simulink model "speed_controller"  (R2023b)
settings: Solver=VariableStepAuto  StartTime=0.0  StopTime=7  RelTol=1e-3
values from neighbouring files (symbols this model uses):
  Kds = 0    [Model_Vars.mat]    (also in pid_tuner.m = sys_pid.Kd)
  Kis = 518.460425454    [Model_Vars.mat]    (also in pid_tuner.m = sys_pid.Ki)
  Kps = 20.988816794    [Model_Vars.mat]    (also in pid_tuner.m = sys_pid.Kp)
undefined symbols (not defined in the file or in its folder): plecs, STire
libraries: nesl_utility x6, fl_lib x5, sdl_lib x3, slpidlib x1, vehdynlibtire x1
settings Model: Creator=jaz43  LastModifiedBy=jaz43
settings SolverCC: InitialStep=.0001  MaxConsecutiveMinStep=100
settings DebuggingCC: AlgebraicLoopMsg=none

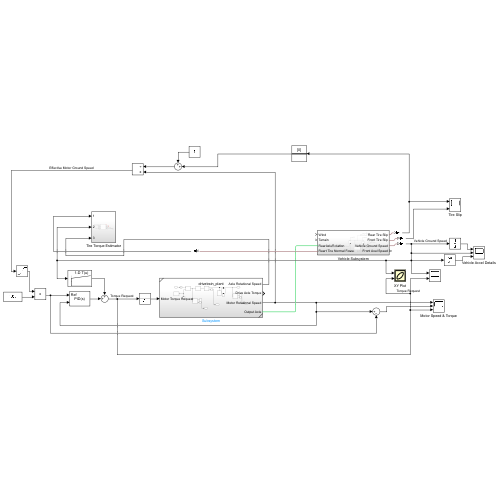
[thumbnail: Simulink's stored preview of the top-level diagram]
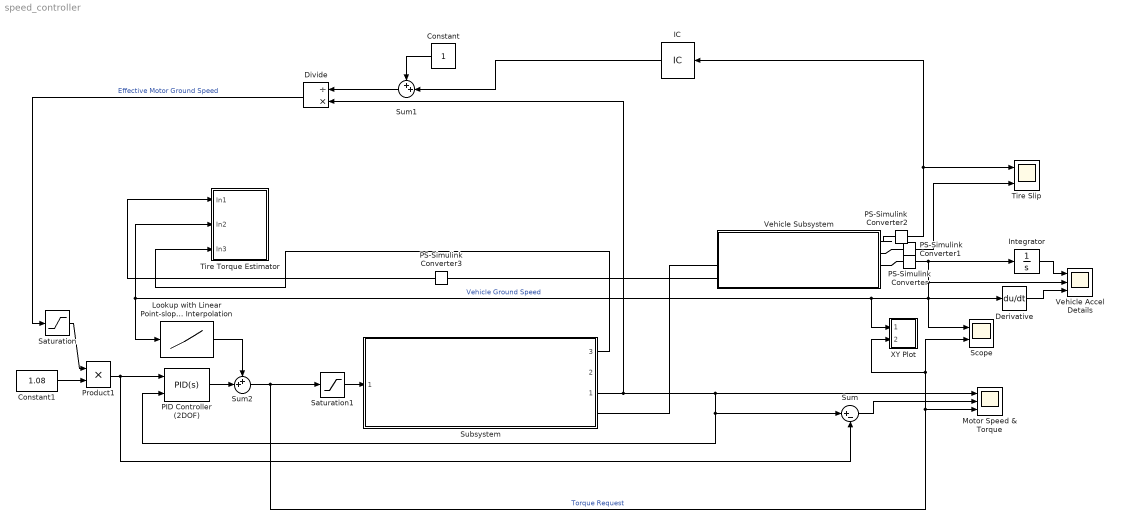
== system speed_controller ==
  Constant : Constant
  Constant1 : Constant  Value=1.08
  Derivative : Derivative
  Divide : Product  Inputs=/*
  IC : InitialCondition  Value=0
  Integrator : Integrator
  Lookup with Linear Point-slope Interpolation : Lookup_n-D  NumberOfTableDimensions=1  BreakpointsForDimension1=[0;0.02;0.05;0.1;0.5;60]  Table=[185;185;185;200;210;218]  InternalRulePriority=Speed  RndMeth=Simplest
  Motor Speed & Torque : Scope  NumInputPorts=3
  PID Controller (2DOF) : slpidlib/PID Controller (2DOF)  Controller=PID  Form=Parallel  TimeDomain=Continuous-time  UseExternalTs=off  SampleTime=-1  IntegratorMethod=Forward Euler  FilterMethod=Forward Euler  ControllerParametersSource=internal  P=Kps  I=Kis  UseKiTs=off  D=Kds  N=0  UseFilter=on  b=1  c=1  TunerSelectOption=Transfer Function Based (PID Tuner App)  InitialConditionSource=internal  InitialConditionForIntegrator=0  InitialConditionForFilter=0  DifferentiatorICPrevScaledInput=0  ExternalReset=none  TrackingMode=off  Kt=1  LimitOutput=off  SatLimitsSource=internal  UpperSaturationLimit=inf  LowerSaturationLimit=-inf  LinearizeAsGain=on  AntiWindupMode=none  Kb=1  LimitIntegrator=on  UpperIntegratorSaturationLimit=20  LowerIntegratorSaturationLimit=-20  POutMin=[]  POutMax=[]  IOutMin=[]  IOutMax=[]  DOutMin=[]  DOutMax=[]  NOutMin=[]  NOutMax=[]  bOutMin=[]  bOutMax=[]  cOutMin=[]  cOutMax=[]  SumOutMin=[]  SumOutMax=[]  SaturationOutMin=[]  SaturationOutMax=[]  PParamMin=[]  PParamMax=[]  IParamMin=[]  IParamMax=[]  DParamMin=[]  DParamMax=[]  NParamMin=[]  NParamMax=[]  bParamMin=[]  bParamMax=[]  cParamMin=[]  cParamMax=[]  KbParamMin=[]  KbParamMax=[]  KtParamMin=[]  KtParamMax=[]  KbOutMin=[]  KbOutMax=[]  KtOutMin=[]  KtOutMax=[]  IntegratorOutMin=[]  IntegratorOutMax=[]  FilterOutMin=[]  FilterOutMax=[]  SumI1OutMin=[]  SumI1OutMax=[]  SumI2OutMin=[]  SumI2OutMax=[]  SumI3OutMin=[]  SumI3OutMax=[]  SumI4OutMin=[]  SumI4OutMax=[]  SumDOutMin=[]  SumDOutMax=[]  Sum1OutMin=[]  Sum1OutMax=[]  Sum2OutMin=[]  Sum2OutMax=[]  Sum3OutMin=[]  Sum3OutMax=[]  DifferentiatorOutMin=[]  DifferentiatorOutMax=[]  FilterDiffOutCoefMin=[]  FilterDiffOutCoefMax=[]  ReciprocalOutMin=[]  ReciprocalOutMax=[]  SumDenOutMin=[]  SumDenOutMax=[]  SumNumOutMin=[]  SumNumOutMax=[]  DivideOutMin=[]  DivideOutMax=[]  UdiffTsProdOutMin=[]  UdiffTsProdOutMax=[]  NTsProdOutMin=[]  NTsProdOutMax=[]  UintegralTsProdOutMin=[]  UintegralTsProdOutMax=[]  UngainTsProdOutMin=[]  UngainTsProdOutMax=[]  ClampingZeroOutDataTypeStr=Inherit: Inherit via back propagation  ClampingZeroOutMin=[]  ClampingZeroOutMax=[]  FilterDenConstantOutDataTypeStr=Inherit: Inherit via back propagation  FilterDenConstantOutMin=[]  FilterDenConstantOutMax=[]  PCopyOutDataTypeStr=Inherit: Inherit via back propagation  PCopyOutMin=[]  PCopyOutMax=[]  NCopyOutDataTypeStr=Inherit: Inherit via back propagation  NCopyOutMin=[]  NCopyOutMax=[]  IntegratorContinuousStateAttributes=''  IntegratorStateMustResolveToSignalObject=off  IntegratorRTWStateStorageClass=Auto  FilterContinuousStateAttributes=''  FilterStateMustResolveToSignalObject=off  FilterRTWStateStorageClass=Auto  ParallelPVariant=InternalParameters  IdealPVariant=Disabled  IVariant=InternalParameters  DVariant=InternalParameters  bVariant=InternalParameters  cVariant=InternalParameters  IntegratorVariant=Continuous  SatVariant=Disabled  AWVariant=Passthrough  PCopyVariant=Disabled  TRVariant=Disabled  FdbkBlocksVariant=Forward  IdealPFdbkVariant=Disabled  SatFdbkVariant=Disabled  DerivativeFilterVariant=ContFilter  NVariant=InternalParameters  NCopyVariant=Disabled  FilterICVariant=InternalICsFilter  IntegratorICVariant=InternalICs  ExternalResetVariant=Disabled  TRSumVariant=Passthrough  SumFdbkVariant=Disabled  SumVariant=Sum_PID  TsampFilterVariant=InternalTs  TsampNgainVariant=Passthrough  TsampIntegralVariant=Disabled_SignalSpec  ExternalSaturationOutDataTypeStr=Inherit: Same as second input
  PS-Simulink Converter : nesl_utility/PS-Simulink Converter  PhysicalDomain=network_engine_domain  SubClassName=ps_output  LeftPortType=input  RightPortType=output  PseudoPeriodic=off  Frequencies=[]  VectorFormat=inherit  Unit=m/s  AffineConversion=off
  PS-Simulink Converter1 : nesl_utility/PS-Simulink Converter  PhysicalDomain=network_engine_domain  SubClassName=ps_output  LeftPortType=input  RightPortType=output  PseudoPeriodic=off  Frequencies=[]  VectorFormat=inherit  Unit=inherit  AffineConversion=off
  PS-Simulink Converter2 : nesl_utility/PS-Simulink Converter  PhysicalDomain=network_engine_domain  SubClassName=ps_output  LeftPortType=input  RightPortType=output  PseudoPeriodic=off  Frequencies=[]  VectorFormat=inherit  Unit=inherit  AffineConversion=off
  PS-Simulink Converter3 : nesl_utility/PS-Simulink Converter  PhysicalDomain=network_engine_domain  SubClassName=ps_output  LeftPortType=input  RightPortType=output  PseudoPeriodic=off  Frequencies=[]  VectorFormat=inherit  Unit=N  AffineConversion=off
  Product1 : Product
  Saturation : Saturate  UpperLimit=10000  LowerLimit=.2
  Saturation1 : Saturate  UpperLimit=230  LowerLimit=-15
  Scope : Scope  NumInputPorts=2
  Subsystem : Subsystem  ReferencedSubsystem=drivetrain_plant
      settings: PortSchema="{\"entries\":[{\"content\":{\"sides\":[{\"content\":{\"connectorIds\":[\"In1\"]},\"type\":\"ConnectorPlacement.EquallySpacedRectSide\",\"uuid\":\"fd89c741-3730-40e8-897c-6a9596430380\"},{\"content\":{\"connectorIds\":[\"Out3\",\"Out2\",\"Out1\",\"RConn1\"],\"side\":\"RIGHT\"},\"type\":\"ConnectorPlacement.EquallySpacedRectSide\",\"uuid\":\"e89eb803-7163-4d37-b99f-28b08d4d828e\"},{\"content\":{\"side\":\"TOP\"},\"type\":\"ConnectorPlacement.EquallySpacedRectSide\",\"uuid\":\"f6f95d47-8b04-417b-a055-58bf5cd7e8eb\"}]},\"type\":\"ConnectorPlacement.EquallySpacedConnector\",\"uuid\":\"a2ebceaa-6fc6-457a-8fcb-4683c2947838\"}],\"packageUris\":[\"http://schema.mathworks.com/mf0/Connector/R2020b\"],\"version\":\"1.0\"}"
  Sum : Sum  Inputs=|+-
  Sum1 : Sum  Inputs=++|
  Sum2 : Sum  Inputs=++|
  Tire Slip : Scope  NumInputPorts=2
  Tire Torque Estimator : Subsystem
  Vehicle Accel Details : Scope  NumInputPorts=3
  Vehicle Subsystem : Subsystem
  XY Plot : Subsystem  LoadFcn=plecs('sl', 317);  InitFcn=plecs('sl', 314);  StartFcn=plecs('sl', 308);  StopFcn=plecs('sl', 309);  mask{Settings=<binary blob, 624 chars, not shown>}
      mask init:
      | plecs('sl', 315);
      settings: CopyFcn=plecs('sl', 318);  DeleteFcn=plecs('sl', 305);  UndoDeleteFcn=plecs('sl', 306);  PreSaveFcn=plecs('sl', 311);  NameChangeFcn=plecs('sl', 310);  DestroyFcn=plecs('sl', 307);  OpenFcn=plecs('sl', 302);  ErrorFcn=plerrorfcn
      mask Display:
      | plot([0.05 0.95 0.95 0.05 0.05], [0.95 0.95 0.05 0.05 0.95])
      | plot(0.5+sin((0:0.2:2)*pi)*0.3, 0.5+sin((0:0.2:2)*pi + pi/4)*0.3);
  wires:
  Sum/1 -> Motor Speed & Torque/2
  PS-Simulink Converter2/1 -> IC/1, Tire Slip/1
  PS-Simulink Converter1/1 -> Tire Slip/2
  Integrator/1 -> Vehicle Accel Details/1
  Derivative/1 -> Vehicle Accel Details/3
  Subsystem/1 -> Divide/2, PID Controller (2DOF)/2, Sum/1, Motor Speed & Torque/1
  Sum1/1 -> Divide/1
  Constant/1 -> Sum1/1
  Constant1/1 -> Product1/2
  Divide/1 -> Saturation/1  "Effective Motor Ground Speed"
  Saturation/1 -> Product1/1
  Sum2/1 -> Saturation1/1, XY Plot/2(2), Scope/2, Motor Speed & Torque/3  "Torque Request"
  PID Controller (2DOF)/1 -> Sum2/2
  IC/1 -> Sum1/2
  Product1/1 -> PID Controller (2DOF)/1, Sum/2
  PS-Simulink Converter/1 -> Derivative/1, Scope/1, XY Plot/1(1), Lookup with Linear Point-slope Interpolation/1, Tire Torque Estimator/2(In2), Vehicle Accel Details/2, Integrator/1  "Vehicle Ground Speed"
  PS-Simulink Converter3/1 -> Tire Torque Estimator/1(In1)
  Subsystem/3 -> Tire Torque Estimator/3(In3)
  Lookup with Linear Point-slope Interpolation/1 -> Sum2/1
  Saturation1/1 -> Subsystem/1
  connections:
  Subsystem/RConn1 -- Vehicle Subsystem/LConn3
  Vehicle Subsystem/RConn3 -- PS-Simulink Converter/LConn1
  PS-Simulink Converter1/LConn1 -- Vehicle Subsystem/RConn2
  Vehicle Subsystem/RConn1 -- PS-Simulink Converter2/LConn1
  Vehicle Subsystem/LConn4 -- PS-Simulink Converter3/LConn1

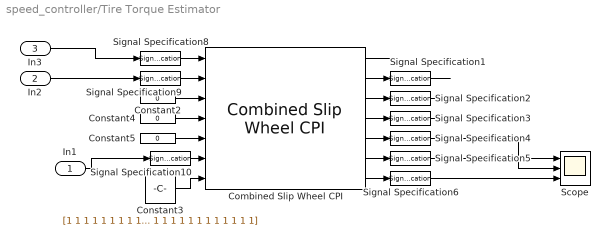
== system speed_controller/Tire Torque Estimator ==
  In1 : Inport
  In2 : Inport  Port=2
  In3 : Inport  Port=3
  Combined Slip Wheel CPI : vehdynlibtire/Combined Slip Wheel CPI  tireType=External file  tireParamSet=C:\Users\jaz43\Documents\2024\Projects\FSAE-LC\Simulink Car Model\testSimscapeCarModel\newtiremodel.tir  TireSide=Left  TirePrs=96526.6  extTirePrs=off  TireIO=CPI  plySteer=off  turnslip=off  PRESMAX=413685.6  PRESMIN=0  FZMAX=100000  FZMIN=0  VXLOW=1  KPUMAX=10  KPUMIN=-10  ALPMAX=0.523598775598299  ALPMIN=-0.523598775598299  CAMMAX=0.174532925199433  CAMMIN=-0.174532925199433  LONGVL=10  tyreside='Right'  FxRelFreqLwrLim=100*pi  FyRelFreqLwrLim=200*pi  MyRelFreqLwrLim=200*pi  omegao=0  br=1e-3  UNLOADED_RADIUS=0.3  NOMPRES=84000  FNOMIN=1500  WIDTH=0.2  RIM_RADIUS=0.2286  ASPECT_RATIO=3.5/6.9  MASS=.1  IYY=1.084  GRAVITY=-9.81  zo=0  zdoto=0  BREFF=8.39  DREFF=0.31475  FREFF=0.14694  Q_RE0=1.003  Q_V1=0.000864  Q_V2=0.025807  Q_FZ1=0  Q_FZ2=51.51  Q_FZ3=0  Q_FCX=0  Q_FCY=0  Q_FCY2=0  PFZ1=1  VERTICAL_STIFFNESS=283576.3  VERTICAL_DAMPING=500  BOTTOM_OFFST=0.01  BOTTOM_STIFF=2000000  Q_CAM1=0  Q_CAM2=0  Q_CAM3=0  LONGITUDINAL_STIFFNESS=505632.6  LATERAL_STIFFNESS=219162.7  PCFX1=-0.12193  PCFX2=0  PCFX3=0  PCFY1=-0.17034  PCFY2=0  PCFY3=0  Q_RA1=0.602  Q_RA2=1.024  Q_RB1=1.1137  Q_RB2=-0.09748  PCX1=1.9  PDX1=2  PDX2=-0.01  PDX3=10  PEX1=-1  PEX2=0.3  PEX3=0  PEX4=0  PKX1=20  PKX2=10  PKX3=0  PHX1=0  PHX2=0  PVX1=0  PVX2=0  PPX1=0  PPX2=0  PPX3=0  PPX4=0  RBX1=5  RBX2=5  RBX3=0  RCX1=1  REX1=-1  REX2=-0.1  RHX1=0  QSX1=0  QSX2=1.5  QSX3=0.1  QSX4=0.1  QSX5=0  QSX6=0  QSX7=0.1  QSX8=0  QSX9=0  QSX10=0  QSX11=0  QSX12=0  QSX13=0  QSX14=0  PPMX1=0  PCY1=2  PDY1=0.8  PDY2=-0.05  PDY3=0  PEY1=-0.8  PEY2=-0.6  PEY3=0.1  PEY4=0  PEY5=0  PKY1=-20  PKY2=2  PKY3=0  PKY4=2  PKY5=0  PKY6=0  PKY7=0  PHY1=0  PHY2=0  PVY1=0  PVY2=0  PVY3=0  PVY4=0  PPY1=0.1  PPY2=0.1  PPY3=0  PPY4=0  PPY5=0  RBY1=5  RBY2=2  RBY3=0.02  RBY4=0  RCY1=1  REY1=-0.1  REY2=0.1  RHY1=0  RHY2=0  RVY1=0  RVY2=0  RVY3=0  RVY4=0  RVY5=0  RVY6=0  QSY1=0  QSY2=0  QSY3=0  QSY4=0  QSY5=0  QSY6=0  QSY7=0  QSY8=0  QBZ1=2.2204e-16  QBZ2=0  QBZ3=0  QBZ4=0  QBZ5=0  QBZ6=0  QBZ9=0  QBZ10=0  QCZ1=0.1  QDZ1=0.1  QDZ2=0  QDZ3=0  QDZ4=0  QDZ6=0  QDZ7=0  QDZ8=0  QDZ9=0  QDZ10=0  QDZ11=0  QEZ1=0  QEZ2=0  QEZ3=0  QEZ4=0  QEZ5=0  QHZ1=0  QHZ2=0  QHZ3=0  QHZ4=0  PPZ1=0  PPZ2=0  SSZ1=0  SSZ2=0  SSZ3=0  SSZ4=0  PDXP1=0  PDXP2=0  PDXP3=0  PKYP1=0  PDYP1=0  PDYP2=0  PDYP3=0  PDYP4=0  PHYP1=0  PHYP2=0  PHYP3=0  PHYP4=0  PECP1=0  PECP2=0  QDTP1=0  QCRP1=0  QCRP2=0  QBRP1=0  QDRP1=0  QDRP2=0  aMode=2
  Constant2 : Constant  Value=0
  Constant3 : Constant  Value=[1 1 1 1 1 1 1 1 1 1 1 1 1 1 1 1 1 1 1 1 1 1 1 1 1 1 1]
  Constant4 : Constant  Value=0
  Constant5 : Constant  Value=0
  Scope : Scope  NumInputPorts=3
  Signal Specification{1..6,8..10} (9 alike) : SignalSpecification  Dimensions=1
  wires:
  Signal Specification4/1 -> Scope/2
  Signal Specification1/1 -> ?
  Signal Specification6/1 -> Scope/3
  Combined Slip Wheel CPI/3 -> Signal Specification2/1
  Combined Slip Wheel CPI/5 -> Signal Specification4/1
  Constant2/1 -> Combined Slip Wheel CPI/3
  Constant5/1 -> Combined Slip Wheel CPI/5
  Combined Slip Wheel CPI/2 -> Signal Specification1/1
  Signal Specification9/1 -> Combined Slip Wheel CPI/2
  Combined Slip Wheel CPI/6 -> Signal Specification5/1
  Signal Specification5/1 -> Scope/1
  Constant3/1 -> Combined Slip Wheel CPI/7
  Signal Specification8/1 -> Combined Slip Wheel CPI/1
  Constant4/1 -> Combined Slip Wheel CPI/4
  Combined Slip Wheel CPI/7 -> Signal Specification6/1
  Combined Slip Wheel CPI/1 -> ?
  Combined Slip Wheel CPI/4 -> Signal Specification3/1
  Signal Specification10/1 -> Combined Slip Wheel CPI/6
  In2/1 -> Signal Specification9/1
  In1/1 -> Signal Specification10/1
  In3/1 -> Signal Specification8/1
  Signal Specification3/1 -> ?
  Signal Specification2/1 -> ?

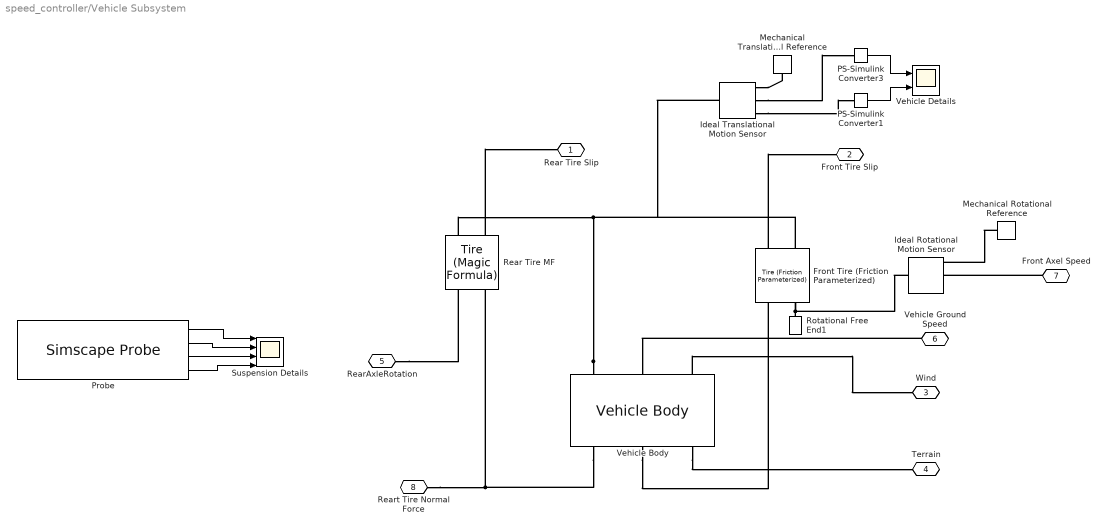
== system speed_controller/Vehicle Subsystem ==
  Front Tire (Friction Parameterized) : sdl_lib/Tires & Vehicles/Tire (Friction Parameterized)  r_tire=508 mm  slip_output=sdl.enum.SlipOutput.Relative  friction_model=sdl.enum.friction_model_var.fixed  mu_static=0.9  mu_kinetic=0.7  slip_vector=[0, .02, .06, .15, .6, 1] rad/s  mu_kinetic_vector=[.89, .88, .8, .75, .7, .7]  interp_method=simscape.enum.interpolation.linear  extrap_method=simscape.enum.extrapolation.linear  model_compliance=sdl.enum.compliance.off  stiffness=1e6 N/m  damping=1000 N*s/m  model_inertia=sdl.enum.model_inertia.off  tire_inertia=1 kg*m^2  initial_velocity=0 rad/s  model_resistance=simscape.enum.onoff.off  resistance_model=sdl.enum.RollingResistance.Constant  coeff=0.015  p_tire=250e3 Pa  alpha=-0.003  beta=0.97  coeff_a=84e-4  coeff_b=6.2e-4 s/m  coeff_c=1.6e-4 s^2/m^2  v_thr=0.001 m/s  v_tol=0.01 m/s  F_min=10 N  initial_traction_state=sdl.enum.tireIC.traction
      settings: InternalSimscapePortConfiguration="{\"Bottom\":[],\"Left\":[{\"id\":\"N\",\"label\":\"N\",\"type\":\"input\"},{\"id\":\"A\",\"label\":\"A\",\"type\":\"foundation.mechanical.rotational.rotational\"}],\"Right\":[{\"id\":\"Srel\",\"label\":\"S\",\"type\":\"output\"},{\"id\":\"H\",\"label\":\"H\",\"type\":\"foundation.mechanical.translational.translational\"}],\"Top\":[]}"
  Ideal Rotational Motion Sensor : fl_lib/Mechanical/Mechanical Sensors/Ideal Rotational Motion Sensor  reference=foundation.enum.MeasurementReference.difference  acceleration_port=false  velocity_port=true  position_port=true  wrap_angle=false  offset=0 rad
  Ideal Translational Motion Sensor : fl_lib/Mechanical/Mechanical Sensors/Ideal Translational Motion Sensor  reference=foundation.enum.MeasurementReference.difference  acceleration_port=false  velocity_port=true  position_port=true  offset=0 m
  Mechanical Rotational Reference : fl_lib/Mechanical/Rotational Elements/Mechanical Rotational Reference
  Mechanical Translational Reference : fl_lib/Mechanical/Translational Elements/Mechanical Translational Reference
  PS-Simulink Converter1 : nesl_utility/PS-Simulink Converter  PhysicalDomain=network_engine_domain  SubClassName=ps_output  LeftPortType=input  RightPortType=output  PseudoPeriodic=off  Frequencies=[]  VectorFormat=inherit  Unit=m  AffineConversion=off
  PS-Simulink Converter3 : nesl_utility/PS-Simulink Converter  PhysicalDomain=network_engine_domain  SubClassName=ps_output  LeftPortType=input  RightPortType=output  PseudoPeriodic=off  Frequencies=[]  VectorFormat=inherit  Unit=m/s  AffineConversion=off
  Probe : SimscapeProbe  BoundBlock=63  Variables={NF, NR, suspension_force_f, suspension_force_r}
  Rear Tire MF : sdl_lib/Tires & Vehicles/Tire (Magic Formula)  parameterization=sdl.enum.magic_tire_model.peak  F_z1=3000 N  F_x1=3500 N  kappa1=8  B_m=10  C_m=1.9  D_m=1  E_m=0.97  fz0=STire.VERTICAL.FNOMIN N  p_Cx=STire.LONGITUDINAL_COEFFICIENTS.PCX  p_Dx=STire.LONGITUDINAL_COEFFICIENTS.PDX  p_Ex=STire.LONGITUDINAL_COEFFICIENTS.PEX  p_Kx=STire.LONGITUDINAL_COEFFICIENTS.PKX  p_Hx=STire.LONGITUDINAL_COEFFICIENTS.PHX  p_Vx=STire.LONGITUDINAL_COEFFICIENTS.PVX  rolling_radius_model=sdl.enum.RollingRadiusParameterization.MagicFormula  r_e=508 mm  r_0=STire.DIMENSION.UNLOADED_RADIUS m  breff=STire.VERTICAL.BREFF  dreff=STire.VERTICAL.DREFF  freff=STire.VERTICAL.FREFF  q_re0=STire.VERTICAL.Q_RE0  q_v1=STire.VERTICAL.Q_V1  longvl=STire.MODEL.LONGVL m/s  cz=STire.VERTICAL.VERTICAL_STIFFNESS N/m  model_resistance=true  resistance_model=sdl.enum.rollingResistanceParameterization.constant  coeff=0.015  p_tire=STire.OPERATING_CONDITIONS.INFLPRES Pa  alpha=-0.003  beta=0.97  coeff_a=84e-4  coeff_b=6.2e-4 s/m  coeff_c=1.6e-4 s^2/m^2  p_tire0=STire.OPERATING_CONDITIONS.NOMPRES Pa  fz0_resistance=STire.VERTICAL.FNOMIN N  vH0=STire.MODEL.LONGVL m/s  q_Sy=STire.ROLLING_COEFFICIENTS.QSY  v_thr=0.001 m/s  enable_scaling_coefficients=true  lfzO=STire.SCALING_COEFFICIENTS.LFZO  lcx=STire.SCALING_COEFFICIENTS.LCX  lmux=STire.SCALING_COEFFICIENTS.LMUX  lex=STire.SCALING_COEFFICIENTS.LEX  lkx=STire.SCALING_COEFFICIENTS.LKX  lhx=STire.SCALING_COEFFICIENTS.LHX  lvx=STire.SCALING_COEFFICIENTS.LVX  lmy=STire.SCALING_COEFFICIENTS.LMY  model_compliance=sdl.enum.compliance.off  stiffness=STire.STRUCTURAL.LONGITUDINAL_STIFFNESS N/m  damping=STire.STRUCTURAL.DAMP_LONG * sqrt(STire.INERTIA.MASS * STire.VERTICAL.FNOMIN / STire.DIMENSION.UNLOADED_RADIUS) N*s/m  model_inertia=sdl.enum.model_inertia.off  inertia=STire.INERTIA.IYY kg*m^2  initial_velocity=0 rad/s  vxlow=0.00001 m/s  v_tr_thr=0.1 m/s  kpumin=-10  kpumax=10
  Rotational Free End1 : fl_lib/Mechanical/Rotational Elements/Rotational Free End  w_specify=off  w_priority=None  w=0 rad/s  w_nominal_specify=off  w_nominal_unit=rad/s  w_nominal_value=1
  Suspension Details : Scope  NumInputPorts=4
  Vehicle Body : sdl_lib/Tires & Vehicles/Vehicle Body  mass=307 kg  n_w=2  x_f=864.45 mm  x_r=665.55 mm  y_c=330 mm  mass_var=simscape.enum.onoff.off  g=9.81 m/s^2  liftoff_warning=simscape.enum.onoff.off  area=3 m^2  Cd=0.4  rho=1.18 kg/m^3  model_pitch=simscape.enum.onoff.on  inertia=500 kg*m^2  suspension_model=sdl.enum.linearTLU.linear  k_f=400*1000 N/m  b_f=1e4 N*s/m  k_r=400*1000 N/m  b_r=1e4 N*s/m  k_f_TLU=[-2000, -1000, 0, 1000, 2000] N  x_f_TLU=[-.4, -.2, 0, .2, .4] m  b_f_TLU=[-200, -100, 0, 100, 200] N  v_f_TLU=[-4, -2, 0, 2, 4] m/s  k_r_TLU=[-2000, -1000, 0, 1000, 2000] N  x_r_TLU=[-.4, -.2, 0, .2, .4] m  b_r_TLU=[-200, -100, 0, 100, 200] N  v_r_TLU=[-4, -2, 0, 2, 4] m/s  interp_method=simscape.enum.interpolation.linear  extrap_method=simscape.enum.extrapolation.linear  model_hardstop=simscape.enum.onoff.off  upper_bound_f=.25 m  lower_bound_f=-.25 m  stop_k_f=1e6 N/m  stop_b_f=150 N*s/m  upper_bound_r=.25 m  lower_bound_r=-.25 m  stop_k_r=1e6 N/m  stop_b_r=150 N*s/m  initial_pitch=0 rad  initial_pitch_rate=0 rad/s  v_specify=off  v_priority=High  v=0 m/s  v_nominal_specify=off  v_nominal_unit=m/s  v_nominal_value=1
  Vehicle Details : Scope  NumInputPorts=2
  Rear Tire Slip : PMIOPort  Side=Right
  Front Tire Slip : PMIOPort  Port=2  Side=Right
  Wind : PMIOPort  Port=3  Side=Left
  Terrain : PMIOPort  Port=4  Side=Left
  RearAxleRotation : PMIOPort  Port=5  Side=Left
  Vehicle Ground Speed : PMIOPort  Port=6  Side=Right
  Front Axel Speed : PMIOPort  Port=7  Side=Right
  Reart Tire Normal Force : PMIOPort  Port=8  Side=Left
  wires:
  PS-Simulink Converter3/1 -> Vehicle Details/1
  PS-Simulink Converter1/1 -> Vehicle Details/2
  Probe/1 -> Suspension Details/1
  Probe/2 -> Suspension Details/2
  Probe/3 -> Suspension Details/3
  Probe/4 -> Suspension Details/4
  connections:
  RearAxleRotation/RConn1 -- Rear Tire MF/LConn2
  Vehicle Body/LConn1 -- Rear Tire MF/RConn2 -- Ideal Translational Motion Sensor/LConn1 -- Front Tire (Friction Parameterized)/RConn2
  Vehicle Body/LConn3 -- Wind/RConn1
  Vehicle Body/RConn3 -- Terrain/RConn1
  Vehicle Body/RConn1 -- Reart Tire Normal Force/RConn1 -- Rear Tire MF/LConn1
  Rotational Free End1/LConn1 -- Ideal Rotational Motion Sensor/LConn1 -- Front Tire (Friction Parameterized)/LConn2
  Vehicle Body/RConn2 -- Front Tire (Friction Parameterized)/LConn1
  Front Tire (Friction Parameterized)/RConn1 -- Front Tire Slip/RConn1
  Rear Tire MF/RConn1 -- Rear Tire Slip/RConn1
  Ideal Translational Motion Sensor/RConn1 -- Mechanical Translational Reference/LConn1
  Ideal Translational Motion Sensor/RConn2 -- PS-Simulink Converter3/LConn1
  Ideal Translational Motion Sensor/RConn3 -- PS-Simulink Converter1/LConn1
  Vehicle Ground Speed/RConn1 -- Vehicle Body/LConn2
  Front Axel Speed/RConn1 -- Ideal Rotational Motion Sensor/RConn2
  Mechanical Rotational Reference/LConn1 -- Ideal Rotational Motion Sensor/RConn1

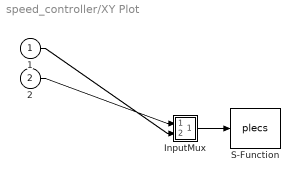
== system speed_controller/XY Plot ==
  1 : Inport
  2 : Inport  Port=2
  " InputMux " : Subsystem
      mask Display: disp('Mux')
  " S-Function " : S-Function  FunctionName=plecs  SFunctionDeploymentMode=off  EnableBusSupport=off
  wires:
  2/1 -> " InputMux "/1(In1)
  1/1 -> " InputMux "/2(In2)
  " InputMux "/1(Out) -> " S-Function "/1

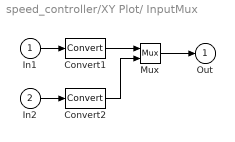
== system speed_controller/XY Plot/ InputMux  ==
  In1 : Inport
  In2 : Inport  Port=2
  Convert1 : DataTypeConversion
  Convert2 : DataTypeConversion
  Mux : Mux  Inputs=2
  Out : Outport
  wires:
  Convert2/1 -> Mux/2
  In2/1 -> Convert2/1
  Convert1/1 -> Mux/1
  In1/1 -> Convert1/1
  Mux/1 -> Out/1
